simulink model "problem5"  (R2020b)
settings: Solver=VariableStepAuto  StartTime=0.0  StopTime=10.0  RelTol=1e-3
PreLoadFcn:
  | R=10;
  | C=10^(-6);
settings Model: Creator=Sayan  LastModifiedBy=Sayan

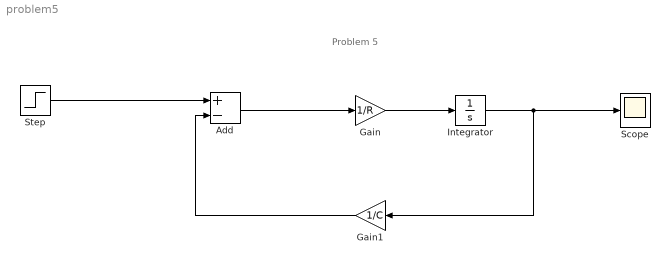
== system problem5 ==
  note: Problem 5
  Add : Sum  Inputs=+-
  Gain : Gain  Gain=1/R
  Gain1 : Gain  Gain=1/C
  Integrator : Integrator
  Scope : Scope
  Step : Step  Before=15  SampleTime=0
  wires:
  Gain1/1 -> Add/2
  Gain/1 -> Integrator/1
  Add/1 -> Gain/1
  Step/1 -> Add/1
  Integrator/1 -> Scope/1, Gain1/1
